simulink model "walkingRobotRL3D"  (R2020b)
settings: Solver=ode23t  StartTime=0.0  StopTime=Tf  RelTol=1e-2  EnableMultiTasking=on
PreLoadFcn:
  | robotParametersRL
undefined symbols (not defined in the file): agent, ankleD_pitch_jointMAX, ankleD_pitch_jointMIN, ankleD_roll_jointMAX, ankleD_roll_jointMIN, ankleI_pitch_jointMAX, ankleI_pitch_jointMIN, ankleI_roll_jointMAX, ankleI_roll_jointMIN, getSampleTime, height_plane, hipD_pitch_jointMAX, hipD_pitch_jointMIN, hipD_roll_jointMAX, hipD_roll_jointMIN, hipI_pitch_jointMAX, hipI_pitch_jointMIN, hipI_roll_jointMAX, hipI_roll_jointMIN, init_angs_L, init_angs_R, init_height, joint_damping, joint_limit_damping, joint_limit_stiffness, joint_stiffness, kneeD_jointMAX, kneeD_jointMIN, kneeI_jointMAX, kneeI_jointMIN, lower_leg_I0, lower_leg_length, lower_leg_mass, lower_leg_x, lower_leg_y, muscle_nominal_length, p10_ankleD_roll, plane_x, plane_y, regulator_type, tau, Tf, torso_height, torso_length, torso_offset_x, torso_offset_z, torso_width, torso_x, torso_y, torso_z, Ts, upper_leg_I0, upper_leg_length, upper_leg_mass, upper_leg_x, upper_leg_y, v10_ankleD_pitch, v10_ankleD_roll, v10_ankleI_pitch, v10_ankleI_roll ... (+41)
libraries: sm_lib x222, simulink x183, nesl_utility x130, walkingRobotUtils x69, rllib x2
(part 15 of 24)

== system walkingRobotRL3D/Walking Robot1/Dynamic model of antagonistic PAM actuators/Spring//Damping (Muscles 2)/Getxmax2 ==
  P2 : Inport
  Bar->kPa : Product
  Constant : Constant  Value=100
  Demux : Demux  Outputs=10
  Mux : Mux  Inputs=10
  getMaxStroke : MATLAB Function  TreatAsAtomicUnit=on
  getMaxStroke1 : MATLAB Function  TreatAsAtomicUnit=on
  getMaxStroke2 : MATLAB Function  TreatAsAtomicUnit=on
  getMaxStroke3 : MATLAB Function  TreatAsAtomicUnit=on
  getMaxStroke4 : MATLAB Function  TreatAsAtomicUnit=on
  getMaxStroke5 : MATLAB Function  TreatAsAtomicUnit=on
  getMaxStroke6 : MATLAB Function  TreatAsAtomicUnit=on
  getMaxStroke7 : MATLAB Function  TreatAsAtomicUnit=on
  getMaxStroke8 : MATLAB Function  TreatAsAtomicUnit=on
  getMaxStroke9 : MATLAB Function  TreatAsAtomicUnit=on
  xmax_muscles2 : Outport
  wires:
  Mux/1 -> xmax_muscles2/1
  P2/1 -> Bar->kPa/2
  Bar->kPa/1 -> Demux/1
  Constant/1 -> Bar->kPa/1
  Demux/1 -> getMaxStroke/1(P2)
  Demux/2 -> getMaxStroke1/1(P2)
  Demux/3 -> getMaxStroke2/1(P2)
  Demux/4 -> getMaxStroke3/1(P2)
  Demux/5 -> getMaxStroke4/1(P2)
  Demux/6 -> getMaxStroke5/1(P2)
  Demux/7 -> getMaxStroke6/1(P2)
  Demux/8 -> getMaxStroke7/1(P2)
  Demux/9 -> getMaxStroke8/1(P2)
  Demux/10 -> getMaxStroke9/1(P2)
  getMaxStroke/1(x_max2) -> Mux/1
  getMaxStroke1/1(x_max2) -> Mux/2
  getMaxStroke2/1(x_max2) -> Mux/3
  getMaxStroke3/1(x_max2) -> Mux/4
  getMaxStroke4/1(x_max2) -> Mux/5
  getMaxStroke5/1(x_max2) -> Mux/6
  getMaxStroke6/1(x_max2) -> Mux/7
  getMaxStroke7/1(x_max2) -> Mux/8
  getMaxStroke8/1(x_max2) -> Mux/9
  getMaxStroke9/1(x_max2) -> Mux/10

== system walkingRobotRL3D/Walking Robot2/Dynamic model of antagonistic PAM actuators/Spring//Damping (Muscles 1)/Get_x1_ankleD_pitch ==
  F1_ankleD_pitchl : Inport
  F2_ankleD_pitch : Inport  Port=2
  S_coef : Inport  Port=3
  Add : Sum  Inputs=+--
  Constant : Constant  Value=tau
  Constant1 : Constant
  Constant2 : Constant  Commented=on  Value=-3.9322
  D_coef : Product
  Divide : Product  Inputs=*/
  IC : InitialCondition  Commented=through  Value=-3.9322
  Integrator : Integrator  InitialCondition=x10_ankleD_pitch
  To Workspace : ToWorkspace  Commented=on  VariableName=S1_ankleD_pitch  SaveFormat=Timeseries  SampleTime=-1
  To Workspace1 : ToWorkspace  Commented=on  VariableName=D1_ankleD_pitch  SaveFormat=Timeseries  SampleTime=-1
  x./D : Product
  xS : Product
  x1_ankleD_pitch : Outport
  wires:
  xS/1 -> Add/3
  x./D/1 -> Integrator/1
  Constant/1 -> D_coef/1
  Divide/1 -> x./D/1
  Constant1/1 -> Divide/1
  D_coef/1 -> To Workspace1/1, Divide/2
  Integrator/1 -> x1_ankleD_pitch/1, xS/1
  IC/1 -> xS/2, To Workspace/1, D_coef/2
  F1_ankleD_pitchl/1 -> Add/1
  F2_ankleD_pitch/1 -> Add/2
  S_coef/1 -> IC/1
  Add/1 -> x./D/2

== system walkingRobotRL3D/Walking Robot2/Dynamic model of antagonistic PAM actuators/Spring//Damping (Muscles 1)/Get_x1_ankleD_roll ==
  F1_ankleD_roll : Inport
  F2_ankleD_roll : Inport  Port=2
  S_coef : Inport  Port=3
  Add : Sum  Inputs=+--
  Constant : Constant  Value=tau
  Constant1 : Constant
  Constant2 : Constant  Commented=on  Value=-3.9322
  D_coef : Product
  Divide : Product  Inputs=*/
  IC : InitialCondition  Commented=through  Value=-3.9322
  Integrator : Integrator  InitialCondition=x10_ankleD_roll
  To Workspace : ToWorkspace  Commented=on  VariableName=S1_ankleD_roll  SaveFormat=Timeseries  SampleTime=-1
  To Workspace1 : ToWorkspace  Commented=on  VariableName=D1_ankleD_roll  SaveFormat=Timeseries  SampleTime=-1
  x./D : Product
  xS : Product
  x1_ankleD_roll : Outport
  wires:
  xS/1 -> Add/3
  x./D/1 -> Integrator/1
  Constant/1 -> D_coef/1
  Divide/1 -> x./D/1
  Constant1/1 -> Divide/1
  D_coef/1 -> To Workspace1/1, Divide/2
  Integrator/1 -> x1_ankleD_roll/1, xS/1
  IC/1 -> xS/2, To Workspace/1, D_coef/2
  F1_ankleD_roll/1 -> Add/1
  F2_ankleD_roll/1 -> Add/2
  S_coef/1 -> IC/1
  Add/1 -> x./D/2

== system walkingRobotRL3D/Walking Robot2/Dynamic model of antagonistic PAM actuators/Spring//Damping (Muscles 1)/Get_x1_ankleI_pitch ==
  F1_ankleI_pitch : Inport
  F2_ankleI_pitch : Inport  Port=2
  S_coef : Inport  Port=3
  Add : Sum  Inputs=+--
  Constant : Constant  Value=tau
  Constant1 : Constant
  D_coef : Product
  Divide : Product  Inputs=*/
  Integrator : Integrator  InitialCondition=x10_ankleI_pitch
  x./D : Product
  xS : Product
  x1_ankleI_pitch : Outport
  wires:
  xS/1 -> Add/3
  Add/1 -> x./D/2
  F1_ankleI_pitch/1 -> Add/1
  F2_ankleI_pitch/1 -> Add/2
  Integrator/1 -> x1_ankleI_pitch/1, xS/1
  S_coef/1 -> D_coef/2, xS/2
  x./D/1 -> Integrator/1
  Constant/1 -> D_coef/1
  Divide/1 -> x./D/1
  Constant1/1 -> Divide/1
  D_coef/1 -> Divide/2

== system walkingRobotRL3D/Walking Robot2/Dynamic model of antagonistic PAM actuators/Spring//Damping (Muscles 1)/Get_x1_ankleI_roll ==
  F1_ankleI_roll : Inport
  F2_ankleI_roll : Inport  Port=2
  S_coef : Inport  Port=3
  Add : Sum  Inputs=+--
  Constant : Constant  Value=tau
  Constant1 : Constant
  D_coef : Product
  Divide : Product  Inputs=*/
  Integrator : Integrator  InitialCondition=x10_ankleI_roll
  x./D : Product
  xS : Product
  x1_ankleI_roll : Outport
  wires:
  xS/1 -> Add/3
  Add/1 -> x./D/2
  F1_ankleI_roll/1 -> Add/1
  F2_ankleI_roll/1 -> Add/2
  Integrator/1 -> x1_ankleI_roll/1, xS/1
  S_coef/1 -> D_coef/2, xS/2
  x./D/1 -> Integrator/1
  Constant/1 -> D_coef/1
  Divide/1 -> x./D/1
  Constant1/1 -> Divide/1
  D_coef/1 -> Divide/2

== system walkingRobotRL3D/Walking Robot2/Dynamic model of antagonistic PAM actuators/Spring//Damping (Muscles 1)/Get_x1_hipD_pitch ==
  F1_hipD_pitch : Inport
  F2_hipD_pitch : Inport  Port=2
  S_coef : Inport  Port=3
  Add : Sum  Inputs=+--
  Constant : Constant  Value=tau
  Constant1 : Constant
  D_coef : Product
  Divide : Product  Inputs=*/
  Integrator : Integrator  InitialCondition=x10_hipD_pitch
  x./D : Product
  xS : Product
  x1_hipD_pitch : Outport
  wires:
  xS/1 -> Add/3
  Add/1 -> x./D/2
  F1_hipD_pitch/1 -> Add/1
  F2_hipD_pitch/1 -> Add/2
  Integrator/1 -> x1_hipD_pitch/1, xS/1
  S_coef/1 -> D_coef/2, xS/2
  x./D/1 -> Integrator/1
  Constant/1 -> D_coef/1
  Divide/1 -> x./D/1
  Constant1/1 -> Divide/1
  D_coef/1 -> Divide/2

== system walkingRobotRL3D/Walking Robot2/Dynamic model of antagonistic PAM actuators/Spring//Damping (Muscles 1)/Get_x1_hipD_roll ==
  F1_hipD_roll : Inport
  F2_hipD_roll : Inport  Port=2
  S_coef : Inport  Port=3
  Add : Sum  Inputs=+--
  Constant : Constant  Value=tau
  Constant1 : Constant
  D_coef : Product
  Divide : Product  Inputs=*/
  Integrator : Integrator  InitialCondition=x10_hipD_roll
  x./D : Product
  xS : Product
  x1_hipD_roll : Outport
  wires:
  xS/1 -> Add/3
  Add/1 -> x./D/2
  F1_hipD_roll/1 -> Add/1
  F2_hipD_roll/1 -> Add/2
  Integrator/1 -> x1_hipD_roll/1, xS/1
  S_coef/1 -> D_coef/2, xS/2
  x./D/1 -> Integrator/1
  Constant/1 -> D_coef/1
  Divide/1 -> x./D/1
  Constant1/1 -> Divide/1
  D_coef/1 -> Divide/2

== system walkingRobotRL3D/Walking Robot2/Dynamic model of antagonistic PAM actuators/Spring//Damping (Muscles 1)/Get_x1_hipI_pitch ==
  F1_hipI_pitch : Inport
  F2_hipI_pitch : Inport  Port=2
  S_coef : Inport  Port=3
  Add : Sum  Inputs=+--
  Constant : Constant  Value=tau
  Constant1 : Constant
  D_coef : Product
  Divide : Product  Inputs=*/
  Integrator : Integrator  InitialCondition=x10_hipI_pitch
  x./D : Product
  xS : Product
  x1_hipI_pitch : Outport
  wires:
  xS/1 -> Add/3
  Add/1 -> x./D/2
  F1_hipI_pitch/1 -> Add/1
  F2_hipI_pitch/1 -> Add/2
  Integrator/1 -> x1_hipI_pitch/1, xS/1
  S_coef/1 -> D_coef/2, xS/2
  x./D/1 -> Integrator/1
  Constant/1 -> D_coef/1
  Divide/1 -> x./D/1
  Constant1/1 -> Divide/1
  D_coef/1 -> Divide/2

== system walkingRobotRL3D/Walking Robot2/Dynamic model of antagonistic PAM actuators/Spring//Damping (Muscles 1)/Get_x1_hipI_roll ==
  F1_hipI_roll : Inport
  F2_hipI_roll : Inport  Port=2
  S_coef : Inport  Port=3
  Add : Sum  Inputs=+--
  Constant : Constant  Value=tau
  Constant1 : Constant
  D_coef : Product
  Divide : Product  Inputs=*/
  Integrator : Integrator  InitialCondition=x10_hipI_roll
  x./D : Product
  xS : Product
  x1_hipI_roll : Outport
  wires:
  xS/1 -> Add/3
  Add/1 -> x./D/2
  F1_hipI_roll/1 -> Add/1
  F2_hipI_roll/1 -> Add/2
  Integrator/1 -> x1_hipI_roll/1, xS/1
  S_coef/1 -> D_coef/2, xS/2
  x./D/1 -> Integrator/1
  Constant/1 -> D_coef/1
  Divide/1 -> x./D/1
  Constant1/1 -> Divide/1
  D_coef/1 -> Divide/2

== system walkingRobotRL3D/Walking Robot2/Dynamic model of antagonistic PAM actuators/Spring//Damping (Muscles 1)/Get_x1_kneeD_1 ==
  F1_kneeD : Inport
  F2_kneeD : Inport  Port=2
  S_coef : Inport  Port=3
  Add : Sum  Inputs=+--
  Constant : Constant  Value=tau
  Constant1 : Constant
  D_coef : Product
  Divide : Product  Inputs=*/
  Integrator : Integrator  InitialCondition=x10_kneeD
  x./D : Product
  xS : Product
  x1_kneeD : Outport
  wires:
  xS/1 -> Add/3
  Add/1 -> x./D/2
  F1_kneeD/1 -> Add/1
  F2_kneeD/1 -> Add/2
  Integrator/1 -> x1_kneeD/1, xS/1
  S_coef/1 -> D_coef/2, xS/2
  x./D/1 -> Integrator/1
  Constant/1 -> D_coef/1
  Divide/1 -> x./D/1
  Constant1/1 -> Divide/1
  D_coef/1 -> Divide/2

== system walkingRobotRL3D/Walking Robot2/Dynamic model of antagonistic PAM actuators/Spring//Damping (Muscles 1)/Get_x1_kneeI ==
  F1_kneeI : Inport
  F2_kneeI : Inport  Port=2
  S_coef : Inport  Port=3
  Add : Sum  Inputs=+--
  Constant : Constant  Value=tau
  Constant1 : Constant
  D_coef : Product
  Divide : Product  Inputs=*/
  Integrator : Integrator  InitialCondition=x10_kneeI
  x./D : Product
  xS : Product
  x1_kneeI : Outport
  wires:
  xS/1 -> Add/3
  Add/1 -> x./D/2
  F1_kneeI/1 -> Add/1
  F2_kneeI/1 -> Add/2
  Integrator/1 -> x1_kneeI/1, xS/1
  S_coef/1 -> D_coef/2, xS/2
  x./D/1 -> Integrator/1
  Constant/1 -> D_coef/1
  Divide/1 -> x./D/1
  Constant1/1 -> Divide/1
  D_coef/1 -> Divide/2

== system walkingRobotRL3D/Walking Robot2/Dynamic model of antagonistic PAM actuators/Spring//Damping (Muscles 1)/Getxmax1 ==
  P1 : Inport
  Bar->kPa : Product
  Constant : Constant  Value=100
  Demux : Demux  Outputs=10
  Mux : Mux  Inputs=10
  To Workspace : ToWorkspace  VariableName=xmax1  SaveFormat=Timeseries  SampleTime=-1
  getMaxStroke : MATLAB Function  TreatAsAtomicUnit=on
  getMaxStroke1 : MATLAB Function  TreatAsAtomicUnit=on
  getMaxStroke2 : MATLAB Function  TreatAsAtomicUnit=on
  getMaxStroke3 : MATLAB Function  TreatAsAtomicUnit=on
  getMaxStroke4 : MATLAB Function  TreatAsAtomicUnit=on
  getMaxStroke5 : MATLAB Function  TreatAsAtomicUnit=on
  getMaxStroke6 : MATLAB Function  TreatAsAtomicUnit=on
  getMaxStroke7 : MATLAB Function  TreatAsAtomicUnit=on
  getMaxStroke8 : MATLAB Function  TreatAsAtomicUnit=on
  getMaxStroke9 : MATLAB Function  TreatAsAtomicUnit=on
  xmax_muscles1 : Outport
  wires:
  Mux/1 -> xmax_muscles1/1
  getMaxStroke/1(x_max1) -> To Workspace/1, Mux/1
  P1/1 -> Bar->kPa/2
  Bar->kPa/1 -> Demux/1
  Constant/1 -> Bar->kPa/1
  Demux/1 -> getMaxStroke/1(P1)
  Demux/2 -> getMaxStroke1/1(P1)
  Demux/3 -> getMaxStroke2/1(P1)
  Demux/4 -> getMaxStroke3/1(P1)
  Demux/5 -> getMaxStroke4/1(P1)
  Demux/6 -> getMaxStroke5/1(P1)
  Demux/7 -> getMaxStroke6/1(P1)
  Demux/8 -> getMaxStroke7/1(P1)
  Demux/9 -> getMaxStroke8/1(P1)
  getMaxStroke1/1(x_max1) -> Mux/2
  getMaxStroke2/1(x_max1) -> Mux/3
  getMaxStroke3/1(x_max1) -> Mux/4
  getMaxStroke4/1(x_max1) -> Mux/5
  getMaxStroke5/1(x_max1) -> Mux/6
  getMaxStroke6/1(x_max1) -> Mux/7
  getMaxStroke7/1(x_max1) -> Mux/8
  getMaxStroke8/1(x_max1) -> Mux/9
  Demux/10 -> getMaxStroke9/1(P1)
  getMaxStroke9/1(x_max1) -> Mux/10

== system walkingRobotRL3D/Walking Robot2/Dynamic model of antagonistic PAM actuators/Spring//Damping (Muscles 2)/Get_x2_ankleD_pitch ==
  F1_ankleD_pitch : Inport
  F2_ankleD_pitch : Inport  Port=2
  S2_coef : Inport  Port=3
  Add : Sum  Inputs=-+-
  Constant : Constant  Value=tau
  Constant1 : Constant
  Constant2 : Constant  Commented=on  Value=3.9338
  D_coef : Product
  Divide : Product  Inputs=*/
  IC : InitialCondition  Commented=through  Value=3.9338
  Integrator : Integrator  InitialCondition=x20_ankleD_pitch
  To Workspace : ToWorkspace  Commented=on  VariableName=S2_ankleD_pitch  SaveFormat=Timeseries  SampleTime=-1
  x./D : Product
  xS : Product
  x2_ankleD_pitch : Outport
  wires:
  xS/1 -> Add/3
  Add/1 -> x./D/2
  F1_ankleD_pitch/1 -> Add/1
  F2_ankleD_pitch/1 -> Add/2
  Integrator/1 -> x2_ankleD_pitch/1, xS/1
  x./D/1 -> Integrator/1
  Constant/1 -> D_coef/1
  Divide/1 -> x./D/1
  Constant1/1 -> Divide/1
  IC/1 -> To Workspace/1, D_coef/2, xS/2
  D_coef/1 -> Divide/2
  S2_coef/1 -> IC/1

== system walkingRobotRL3D/Walking Robot2/Dynamic model of antagonistic PAM actuators/Spring//Damping (Muscles 2)/Get_x2_ankleD_roll ==
  F1_ankleD_roll : Inport
  F2_ankleD_roll : Inport  Port=2
  S2_coef : Inport  Port=3
  Add : Sum  Inputs=-+-
  Constant : Constant  Value=tau
  Constant1 : Constant
  Constant2 : Constant  Commented=on  Value=3.9338
  D_coef : Product
  Divide : Product  Inputs=*/
  IC : InitialCondition  Commented=through  Value=3.9338
  Integrator : Integrator  InitialCondition=x20_ankleD_roll
  To Workspace : ToWorkspace  Commented=on  VariableName=S2_ankleD_roll  SaveFormat=Timeseries  SampleTime=-1
  x./D : Product
  xS : Product
  x2_ankleD_roll : Outport
  wires:
  xS/1 -> Add/3
  Add/1 -> x./D/2
  F1_ankleD_roll/1 -> Add/1
  F2_ankleD_roll/1 -> Add/2
  Integrator/1 -> x2_ankleD_roll/1, xS/1
  x./D/1 -> Integrator/1
  Constant/1 -> D_coef/1
  Divide/1 -> x./D/1
  Constant1/1 -> Divide/1
  IC/1 -> To Workspace/1, D_coef/2, xS/2
  D_coef/1 -> Divide/2
  S2_coef/1 -> IC/1

== system walkingRobotRL3D/Walking Robot2/Dynamic model of antagonistic PAM actuators/Spring//Damping (Muscles 2)/Get_x2_ankleI_pitch ==
  F1_ankleI_pitch : Inport
  F2_ankleI_pitch : Inport  Port=2
  S2_coef : Inport  Port=3
  Add : Sum  Inputs=-+-
  Constant : Constant  Value=tau
  Constant1 : Constant
  D_coef : Product
  Divide : Product  Inputs=*/
  Integrator : Integrator  InitialCondition=x20_ankleI_pitch
  x./D : Product
  xS : Product
  x2_ankleI_pitch : Outport
  wires:
  xS/1 -> Add/3
  Add/1 -> x./D/2
  F1_ankleI_pitch/1 -> Add/1
  F2_ankleI_pitch/1 -> Add/2
  Integrator/1 -> x2_ankleI_pitch/1, xS/1
  S2_coef/1 -> D_coef/2, xS/2
  x./D/1 -> Integrator/1
  Constant/1 -> D_coef/1
  Divide/1 -> x./D/1
  Constant1/1 -> Divide/1
  D_coef/1 -> Divide/2

== system walkingRobotRL3D/Walking Robot2/Dynamic model of antagonistic PAM actuators/Spring//Damping (Muscles 2)/Get_x2_ankleI_roll ==
  F1_ankleI_roll : Inport
  F2_ankleI_roll : Inport  Port=2
  S2_coef : Inport  Port=3
  Add : Sum  Inputs=-+-
  Constant : Constant  Value=tau
  Constant1 : Constant
  D_coef : Product
  Divide : Product  Inputs=*/
  Integrator : Integrator  InitialCondition=x20_ankleI_roll
  x./D : Product
  xS : Product
  x2_ankleI_roll : Outport
  wires:
  xS/1 -> Add/3
  Add/1 -> x./D/2
  F1_ankleI_roll/1 -> Add/1
  F2_ankleI_roll/1 -> Add/2
  Integrator/1 -> x2_ankleI_roll/1, xS/1
  S2_coef/1 -> D_coef/2, xS/2
  x./D/1 -> Integrator/1
  Constant/1 -> D_coef/1
  Divide/1 -> x./D/1
  Constant1/1 -> Divide/1
  D_coef/1 -> Divide/2

== system walkingRobotRL3D/Walking Robot2/Dynamic model of antagonistic PAM actuators/Spring//Damping (Muscles 2)/Get_x2_hipD_pitch ==
  F1_hipD_pitch : Inport
  F2_hipD_pitch : Inport  Port=2
  S2_coef : Inport  Port=3
  Add : Sum  Inputs=-+-
  Constant : Constant  Value=tau
  Constant1 : Constant
  D_coef : Product
  Divide : Product  Inputs=*/
  Integrator : Integrator  InitialCondition=x20_hipD_pitch
  x./D : Product
  xS : Product
  x2_hipD_pitch : Outport
  wires:
  xS/1 -> Add/3
  Add/1 -> x./D/2
  F1_hipD_pitch/1 -> Add/1
  F2_hipD_pitch/1 -> Add/2
  Integrator/1 -> x2_hipD_pitch/1, xS/1
  S2_coef/1 -> D_coef/2, xS/2
  x./D/1 -> Integrator/1
  Constant/1 -> D_coef/1
  Divide/1 -> x./D/1
  Constant1/1 -> Divide/1
  D_coef/1 -> Divide/2

== system walkingRobotRL3D/Walking Robot2/Dynamic model of antagonistic PAM actuators/Spring//Damping (Muscles 2)/Get_x2_hipD_roll ==
  F1_hipD_roll : Inport
  F2_hipD_roll : Inport  Port=2
  S2_coef : Inport  Port=3
  Add : Sum  Inputs=-+-
  Constant : Constant  Value=tau
  Constant1 : Constant
  D_coef : Product
  Divide : Product  Inputs=*/
  Integrator : Integrator  InitialCondition=x20_hipD_roll
  x./D : Product
  xS : Product
  x2_hipD_roll : Outport
  wires:
  xS/1 -> Add/3
  Add/1 -> x./D/2
  F1_hipD_roll/1 -> Add/1
  F2_hipD_roll/1 -> Add/2
  Integrator/1 -> x2_hipD_roll/1, xS/1
  S2_coef/1 -> D_coef/2, xS/2
  x./D/1 -> Integrator/1
  Constant/1 -> D_coef/1
  Divide/1 -> x./D/1
  Constant1/1 -> Divide/1
  D_coef/1 -> Divide/2

== system walkingRobotRL3D/Walking Robot2/Dynamic model of antagonistic PAM actuators/Spring//Damping (Muscles 2)/Get_x2_hipI_pitch ==
  F1_hipI_pitch : Inport
  F2_hipI_pitch : Inport  Port=2
  S2_coef : Inport  Port=3
  Add : Sum  Inputs=-+-
  Constant : Constant  Value=tau
  Constant1 : Constant
  D_coef : Product
  Divide : Product  Inputs=*/
  Integrator : Integrator  InitialCondition=x20_hipI_pitch
  x./D : Product
  xS : Product
  x2_hipI_pitch : Outport
  wires:
  xS/1 -> Add/3
  Add/1 -> x./D/2
  F1_hipI_pitch/1 -> Add/1
  F2_hipI_pitch/1 -> Add/2
  Integrator/1 -> x2_hipI_pitch/1, xS/1
  S2_coef/1 -> D_coef/2, xS/2
  x./D/1 -> Integrator/1
  Constant/1 -> D_coef/1
  Divide/1 -> x./D/1
  Constant1/1 -> Divide/1
  D_coef/1 -> Divide/2

== system walkingRobotRL3D/Walking Robot2/Dynamic model of antagonistic PAM actuators/Spring//Damping (Muscles 2)/Get_x2_hipI_roll ==
  F1_hipI_roll : Inport
  F2_hipI_roll : Inport  Port=2
  S2_coef : Inport  Port=3
  Add : Sum  Inputs=-+-
  Constant : Constant  Value=tau
  Constant1 : Constant
  D_coef : Product
  Divide : Product  Inputs=*/
  Integrator : Integrator  InitialCondition=x20_hipI_roll
  x./D : Product
  xS : Product
  x2_hipI_roll : Outport
  wires:
  xS/1 -> Add/3
  Add/1 -> x./D/2
  F1_hipI_roll/1 -> Add/1
  F2_hipI_roll/1 -> Add/2
  Integrator/1 -> x2_hipI_roll/1, xS/1
  S2_coef/1 -> D_coef/2, xS/2
  x./D/1 -> Integrator/1
  Constant/1 -> D_coef/1
  Divide/1 -> x./D/1
  Constant1/1 -> Divide/1
  D_coef/1 -> Divide/2

== system walkingRobotRL3D/Walking Robot2/Dynamic model of antagonistic PAM actuators/Spring//Damping (Muscles 2)/Get_x2_kneeD ==
  F1_kneeD : Inport
  F2_kneeI : Inport  Port=2
  S2_coef : Inport  Port=3
  Add : Sum  Inputs=-+-
  Constant : Constant  Value=tau
  Constant1 : Constant
  D_coef : Product
  Divide : Product  Inputs=*/
  Integrator : Integrator  InitialCondition=x20_kneeD
  x./D : Product
  xS : Product
  x2_kneeD : Outport
  wires:
  xS/1 -> Add/3
  Add/1 -> x./D/2
  F1_kneeD/1 -> Add/1
  F2_kneeI/1 -> Add/2
  Integrator/1 -> x2_kneeD/1, xS/1
  S2_coef/1 -> D_coef/2, xS/2
  x./D/1 -> Integrator/1
  Constant/1 -> D_coef/1
  Divide/1 -> x./D/1
  Constant1/1 -> Divide/1
  D_coef/1 -> Divide/2

== system walkingRobotRL3D/Walking Robot2/Dynamic model of antagonistic PAM actuators/Spring//Damping (Muscles 2)/Get_x2_kneeI ==
  F1_kneeI : Inport
  F2_kneeI : Inport  Port=2
  S2_coef : Inport  Port=3
  Add : Sum  Inputs=-+-
  Constant : Constant  Value=tau
  Constant1 : Constant
  D_coef : Product
  Divide : Product  Inputs=*/
  Integrator : Integrator  InitialCondition=x20_kneeI
  x./D : Product
  xS : Product
  x2_kneeI : Outport
  wires:
  xS/1 -> Add/3
  Add/1 -> x./D/2
  F1_kneeI/1 -> Add/1
  F2_kneeI/1 -> Add/2
  Integrator/1 -> x2_kneeI/1, xS/1
  S2_coef/1 -> D_coef/2, xS/2
  x./D/1 -> Integrator/1
  Constant/1 -> D_coef/1
  Divide/1 -> x./D/1
  Constant1/1 -> Divide/1
  D_coef/1 -> Divide/2

== system walkingRobotRL3D/Walking Robot2/Dynamic model of antagonistic PAM actuators/Spring//Damping (Muscles 2)/Getxmax2 ==
  P2 : Inport
  Bar->kPa : Product
  Constant : Constant  Value=100
  Demux : Demux  Outputs=10
  Mux : Mux  Inputs=10
  getMaxStroke : MATLAB Function  TreatAsAtomicUnit=on
  getMaxStroke1 : MATLAB Function  TreatAsAtomicUnit=on
  getMaxStroke2 : MATLAB Function  TreatAsAtomicUnit=on
  getMaxStroke3 : MATLAB Function  TreatAsAtomicUnit=on
  getMaxStroke4 : MATLAB Function  TreatAsAtomicUnit=on
  getMaxStroke5 : MATLAB Function  TreatAsAtomicUnit=on
  getMaxStroke6 : MATLAB Function  TreatAsAtomicUnit=on
  getMaxStroke7 : MATLAB Function  TreatAsAtomicUnit=on
  getMaxStroke8 : MATLAB Function  TreatAsAtomicUnit=on
  getMaxStroke9 : MATLAB Function  TreatAsAtomicUnit=on
  xmax_muscles2 : Outport
  wires:
  Mux/1 -> xmax_muscles2/1
  P2/1 -> Bar->kPa/2
  Bar->kPa/1 -> Demux/1
  Constant/1 -> Bar->kPa/1
  Demux/1 -> getMaxStroke/1(P2)
  Demux/2 -> getMaxStroke1/1(P2)
  Demux/3 -> getMaxStroke2/1(P2)
  Demux/4 -> getMaxStroke3/1(P2)
  Demux/5 -> getMaxStroke4/1(P2)
  Demux/6 -> getMaxStroke5/1(P2)
  Demux/7 -> getMaxStroke6/1(P2)
  Demux/8 -> getMaxStroke7/1(P2)
  Demux/9 -> getMaxStroke8/1(P2)
  Demux/10 -> getMaxStroke9/1(P2)
  getMaxStroke/1(x_max2) -> Mux/1
  getMaxStroke1/1(x_max2) -> Mux/2
  getMaxStroke2/1(x_max2) -> Mux/3
  getMaxStroke3/1(x_max2) -> Mux/4
  getMaxStroke4/1(x_max2) -> Mux/5
  getMaxStroke5/1(x_max2) -> Mux/6
  getMaxStroke6/1(x_max2) -> Mux/7
  getMaxStroke7/1(x_max2) -> Mux/8
  getMaxStroke8/1(x_max2) -> Mux/9
  getMaxStroke9/1(x_max2) -> Mux/10

== system walkingRobotRL3D/Walking Robot33/DYNAMIC MODEL OF PAM FOR LEFT LEG/Dynamic Model Antagonisitic PAM1/Spring and damping model ==
  F1 : Inport
  F2 : Inport  Port=2
  P1 : Inport  Port=3
  P2 : Inport  Port=4
  Dynamic muscle 2 : Subsystem
  Dynamics muscle 1 : Subsystem
  S(P),D(P) : MATLAB Function  TreatAsAtomicUnit=on
  Unit Delay : UnitDelay  SampleTime=-1  HasFrameUpgradeWarning=on
  Unit Delay1 : UnitDelay  SampleTime=-1  HasFrameUpgradeWarning=on
  Unit Delay2 : UnitDelay  Commented=through  SampleTime=-1  HasFrameUpgradeWarning=on
  Unit Delay3 : UnitDelay  Commented=through  SampleTime=-1  HasFrameUpgradeWarning=on
  x1(m)->x1(%) : Gain  Gain=100/muscle_nominal_length
  x2(m)->x2(%) : Gain  Gain=100/muscle_nominal_length
  x2 : Outport
  x1 : Outport  Port=2
  wires:
  Dynamics muscle 1/1(R1) -> Unit Delay/1
  F1/1 -> Unit Delay2/1
  Dynamic muscle 2/2(x2) -> x2(m)->x2(%)/1
  Dynamics muscle 1/2(x1) -> x1(m)->x1(%)/1
  P1/1 -> S(P),D(P)/1(P1)
  x2(m)->x2(%)/1 -> x2/1
  x1(m)->x1(%)/1 -> x1/1
  F2/1 -> Unit Delay3/1
  P2/1 -> S(P),D(P)/2(P2)
  Unit Delay/1 -> Dynamic muscle 2/2(R1)
  Dynamic muscle 2/1(R2) -> Unit Delay1/1
  Unit Delay1/1 -> Dynamics muscle 1/3(R2)
  Unit Delay2/1 -> Dynamics muscle 1/1(F1)
  Unit Delay3/1 -> Dynamic muscle 2/3(F2)
  S(P),D(P)/2(D1) -> Dynamics muscle 1/4(D1)
  S(P),D(P)/3(S2) -> Dynamic muscle 2/1(S2)
  S(P),D(P)/4(D2) -> Dynamic muscle 2/4(D2)
  S(P),D(P)/1(S1) -> Dynamics muscle 1/2(S1)

== system walkingRobotRL3D/Walking Robot33/DYNAMIC MODEL OF PAM FOR LEFT LEG/Dynamic Model Antagonisitic PAM2/Spring and damping model ==
  F1 : Inport
  F2 : Inport  Port=2
  P1 : Inport  Port=3
  P2 : Inport  Port=4
  Dynamic muscle 2 : Subsystem
  Dynamics muscle 1 : Subsystem
  S(P),D(P) : MATLAB Function  TreatAsAtomicUnit=on
  Unit Delay : UnitDelay  SampleTime=-1  HasFrameUpgradeWarning=on
  Unit Delay1 : UnitDelay  SampleTime=-1  HasFrameUpgradeWarning=on
  Unit Delay2 : UnitDelay  Commented=through  SampleTime=-1  HasFrameUpgradeWarning=on
  Unit Delay3 : UnitDelay  Commented=through  SampleTime=-1  HasFrameUpgradeWarning=on
  x1(m)->x1(%) : Gain  Gain=100/muscle_nominal_length
  x2(m)->x2(%) : Gain  Gain=100/muscle_nominal_length
  x2 : Outport
  x1 : Outport  Port=2
  wires:
  Dynamics muscle 1/1(R1) -> Unit Delay/1
  F1/1 -> Unit Delay2/1
  Dynamic muscle 2/2(x2) -> x2(m)->x2(%)/1
  Dynamics muscle 1/2(x1) -> x1(m)->x1(%)/1
  P1/1 -> S(P),D(P)/1(P1)
  x2(m)->x2(%)/1 -> x2/1
  x1(m)->x1(%)/1 -> x1/1
  F2/1 -> Unit Delay3/1
  P2/1 -> S(P),D(P)/2(P2)
  Unit Delay/1 -> Dynamic muscle 2/2(R1)
  Dynamic muscle 2/1(R2) -> Unit Delay1/1
  Unit Delay1/1 -> Dynamics muscle 1/3(R2)
  Unit Delay2/1 -> Dynamics muscle 1/1(F1)
  Unit Delay3/1 -> Dynamic muscle 2/3(F2)
  S(P),D(P)/2(D1) -> Dynamics muscle 1/4(D1)
  S(P),D(P)/3(S2) -> Dynamic muscle 2/1(S2)
  S(P),D(P)/4(D2) -> Dynamic muscle 2/4(D2)
  S(P),D(P)/1(S1) -> Dynamics muscle 1/2(S1)

== system walkingRobotRL3D/Walking Robot33/DYNAMIC MODEL OF PAM FOR LEFT LEG/Dynamic Model Antagonisitic PAM3/Spring and damping model ==
  F1 : Inport
  F2 : Inport  Port=2
  P1 : Inport  Port=3
  P2 : Inport  Port=4
  Dynamic muscle 2 : Subsystem
  Dynamics muscle 1 : Subsystem
  S(P),D(P) : MATLAB Function  TreatAsAtomicUnit=on
  Unit Delay : UnitDelay  SampleTime=-1  HasFrameUpgradeWarning=on
  Unit Delay1 : UnitDelay  SampleTime=-1  HasFrameUpgradeWarning=on
  Unit Delay2 : UnitDelay  Commented=through  SampleTime=-1  HasFrameUpgradeWarning=on
  Unit Delay3 : UnitDelay  Commented=through  SampleTime=-1  HasFrameUpgradeWarning=on
  x1(m)->x1(%) : Gain  Gain=100/muscle_nominal_length
  x2(m)->x2(%) : Gain  Gain=100/muscle_nominal_length
  x2 : Outport
  x1 : Outport  Port=2
  wires:
  Dynamics muscle 1/1(R1) -> Unit Delay/1
  F1/1 -> Unit Delay2/1
  Dynamic muscle 2/2(x2) -> x2(m)->x2(%)/1
  Dynamics muscle 1/2(x1) -> x1(m)->x1(%)/1
  P1/1 -> S(P),D(P)/1(P1)
  x2(m)->x2(%)/1 -> x2/1
  x1(m)->x1(%)/1 -> x1/1
  F2/1 -> Unit Delay3/1
  P2/1 -> S(P),D(P)/2(P2)
  Unit Delay/1 -> Dynamic muscle 2/2(R1)
  Dynamic muscle 2/1(R2) -> Unit Delay1/1
  Unit Delay1/1 -> Dynamics muscle 1/3(R2)
  Unit Delay2/1 -> Dynamics muscle 1/1(F1)
  Unit Delay3/1 -> Dynamic muscle 2/3(F2)
  S(P),D(P)/2(D1) -> Dynamics muscle 1/4(D1)
  S(P),D(P)/3(S2) -> Dynamic muscle 2/1(S2)
  S(P),D(P)/4(D2) -> Dynamic muscle 2/4(D2)
  S(P),D(P)/1(S1) -> Dynamics muscle 1/2(S1)

== system walkingRobotRL3D/Walking Robot33/DYNAMIC MODEL OF PAM FOR LEFT LEG/Dynamic Model Antagonisitic PAM4/Spring and damping model ==
  F1 : Inport
  F2 : Inport  Port=2
  P1 : Inport  Port=3
  P2 : Inport  Port=4
  Dynamic muscle 2 : Subsystem
  Dynamics muscle 1 : Subsystem
  S(P),D(P) : MATLAB Function  TreatAsAtomicUnit=on
  Unit Delay : UnitDelay  SampleTime=-1  HasFrameUpgradeWarning=on
  Unit Delay1 : UnitDelay  SampleTime=-1  HasFrameUpgradeWarning=on
  Unit Delay2 : UnitDelay  Commented=through  SampleTime=-1  HasFrameUpgradeWarning=on
  Unit Delay3 : UnitDelay  Commented=through  SampleTime=-1  HasFrameUpgradeWarning=on
  x1(m)->x1(%) : Gain  Gain=100/muscle_nominal_length
  x2(m)->x2(%) : Gain  Gain=100/muscle_nominal_length
  x2 : Outport
  x1 : Outport  Port=2
  wires:
  Dynamics muscle 1/1(R1) -> Unit Delay/1
  F1/1 -> Unit Delay2/1
  Dynamic muscle 2/2(x2) -> x2(m)->x2(%)/1
  Dynamics muscle 1/2(x1) -> x1(m)->x1(%)/1
  P1/1 -> S(P),D(P)/1(P1)
  x2(m)->x2(%)/1 -> x2/1
  x1(m)->x1(%)/1 -> x1/1
  F2/1 -> Unit Delay3/1
  P2/1 -> S(P),D(P)/2(P2)
  Unit Delay/1 -> Dynamic muscle 2/2(R1)
  Dynamic muscle 2/1(R2) -> Unit Delay1/1
  Unit Delay1/1 -> Dynamics muscle 1/3(R2)
  Unit Delay2/1 -> Dynamics muscle 1/1(F1)
  Unit Delay3/1 -> Dynamic muscle 2/3(F2)
  S(P),D(P)/2(D1) -> Dynamics muscle 1/4(D1)
  S(P),D(P)/3(S2) -> Dynamic muscle 2/1(S2)
  S(P),D(P)/4(D2) -> Dynamic muscle 2/4(D2)
  S(P),D(P)/1(S1) -> Dynamics muscle 1/2(S1)

== system walkingRobotRL3D/Walking Robot33/DYNAMIC MODEL OF PAM FOR LEFT LEG/Dynamic Model Antagonisitic PAM5/Spring and damping model ==
  F1 : Inport
  F2 : Inport  Port=2
  P1 : Inport  Port=3
  P2 : Inport  Port=4
  Dynamic muscle 2 : Subsystem
  Dynamics muscle 1 : Subsystem
  S(P),D(P) : MATLAB Function  TreatAsAtomicUnit=on
  Unit Delay : UnitDelay  SampleTime=-1  HasFrameUpgradeWarning=on
  Unit Delay1 : UnitDelay  SampleTime=-1  HasFrameUpgradeWarning=on
  Unit Delay2 : UnitDelay  Commented=through  SampleTime=-1  HasFrameUpgradeWarning=on
  Unit Delay3 : UnitDelay  Commented=through  SampleTime=-1  HasFrameUpgradeWarning=on
  x1(m)->x1(%) : Gain  Gain=100/muscle_nominal_length
  x2(m)->x2(%) : Gain  Gain=100/muscle_nominal_length
  x2 : Outport
  x1 : Outport  Port=2
  wires:
  Dynamics muscle 1/1(R1) -> Unit Delay/1
  F1/1 -> Unit Delay2/1
  Dynamic muscle 2/2(x2) -> x2(m)->x2(%)/1
  Dynamics muscle 1/2(x1) -> x1(m)->x1(%)/1
  P1/1 -> S(P),D(P)/1(P1)
  x2(m)->x2(%)/1 -> x2/1
  x1(m)->x1(%)/1 -> x1/1
  F2/1 -> Unit Delay3/1
  P2/1 -> S(P),D(P)/2(P2)
  Unit Delay/1 -> Dynamic muscle 2/2(R1)
  Dynamic muscle 2/1(R2) -> Unit Delay1/1
  Unit Delay1/1 -> Dynamics muscle 1/3(R2)
  Unit Delay2/1 -> Dynamics muscle 1/1(F1)
  Unit Delay3/1 -> Dynamic muscle 2/3(F2)
  S(P),D(P)/2(D1) -> Dynamics muscle 1/4(D1)
  S(P),D(P)/3(S2) -> Dynamic muscle 2/1(S2)
  S(P),D(P)/4(D2) -> Dynamic muscle 2/4(D2)
  S(P),D(P)/1(S1) -> Dynamics muscle 1/2(S1)

== system walkingRobotRL3D/Walking Robot33/DYNAMIC MODEL OF PAM FOR RIGHT LEG/Dynamic Model Antagonisitic PAM1/Spring and damping model ==
  F1 : Inport
  F2 : Inport  Port=2
  P1 : Inport  Port=3
  P2 : Inport  Port=4
  Dynamic muscle 2 : Subsystem
  Dynamics muscle 1 : Subsystem
  S(P),D(P) : MATLAB Function  TreatAsAtomicUnit=on
  Unit Delay : UnitDelay  SampleTime=-1  HasFrameUpgradeWarning=on
  Unit Delay1 : UnitDelay  SampleTime=-1  HasFrameUpgradeWarning=on
  Unit Delay2 : UnitDelay  Commented=through  SampleTime=-1  HasFrameUpgradeWarning=on
  Unit Delay3 : UnitDelay  Commented=through  SampleTime=-1  HasFrameUpgradeWarning=on
  x1(m)->x1(%) : Gain  Gain=100/muscle_nominal_length
  x2(m)->x2(%) : Gain  Gain=100/muscle_nominal_length
  x2 : Outport
  x1 : Outport  Port=2
  wires:
  Dynamics muscle 1/1(R1) -> Unit Delay/1
  F1/1 -> Unit Delay2/1
  Dynamic muscle 2/2(x2) -> x2(m)->x2(%)/1
  Dynamics muscle 1/2(x1) -> x1(m)->x1(%)/1
  P1/1 -> S(P),D(P)/1(P1)
  x2(m)->x2(%)/1 -> x2/1
  x1(m)->x1(%)/1 -> x1/1
  F2/1 -> Unit Delay3/1
  P2/1 -> S(P),D(P)/2(P2)
  Unit Delay/1 -> Dynamic muscle 2/2(R1)
  Dynamic muscle 2/1(R2) -> Unit Delay1/1
  Unit Delay1/1 -> Dynamics muscle 1/3(R2)
  Unit Delay2/1 -> Dynamics muscle 1/1(F1)
  Unit Delay3/1 -> Dynamic muscle 2/3(F2)
  S(P),D(P)/2(D1) -> Dynamics muscle 1/4(D1)
  S(P),D(P)/3(S2) -> Dynamic muscle 2/1(S2)
  S(P),D(P)/4(D2) -> Dynamic muscle 2/4(D2)
  S(P),D(P)/1(S1) -> Dynamics muscle 1/2(S1)

== system walkingRobotRL3D/Walking Robot33/DYNAMIC MODEL OF PAM FOR RIGHT LEG/Dynamic Model Antagonisitic PAM2/Spring and damping model ==
  F1 : Inport
  F2 : Inport  Port=2
  P1 : Inport  Port=3
  P2 : Inport  Port=4
  Dynamic muscle 2 : Subsystem
  Dynamics muscle 1 : Subsystem
  S(P),D(P) : MATLAB Function  TreatAsAtomicUnit=on
  Unit Delay : UnitDelay  SampleTime=-1  HasFrameUpgradeWarning=on
  Unit Delay1 : UnitDelay  SampleTime=-1  HasFrameUpgradeWarning=on
  Unit Delay2 : UnitDelay  Commented=through  SampleTime=-1  HasFrameUpgradeWarning=on
  Unit Delay3 : UnitDelay  Commented=through  SampleTime=-1  HasFrameUpgradeWarning=on
  x1(m)->x1(%) : Gain  Gain=100/muscle_nominal_length
  x2(m)->x2(%) : Gain  Gain=100/muscle_nominal_length
  x2 : Outport
  x1 : Outport  Port=2
  wires:
  Dynamics muscle 1/1(R1) -> Unit Delay/1
  F1/1 -> Unit Delay2/1
  Dynamic muscle 2/2(x2) -> x2(m)->x2(%)/1
  Dynamics muscle 1/2(x1) -> x1(m)->x1(%)/1
  P1/1 -> S(P),D(P)/1(P1)
  x2(m)->x2(%)/1 -> x2/1
  x1(m)->x1(%)/1 -> x1/1
  F2/1 -> Unit Delay3/1
  P2/1 -> S(P),D(P)/2(P2)
  Unit Delay/1 -> Dynamic muscle 2/2(R1)
  Dynamic muscle 2/1(R2) -> Unit Delay1/1
  Unit Delay1/1 -> Dynamics muscle 1/3(R2)
  Unit Delay2/1 -> Dynamics muscle 1/1(F1)
  Unit Delay3/1 -> Dynamic muscle 2/3(F2)
  S(P),D(P)/2(D1) -> Dynamics muscle 1/4(D1)
  S(P),D(P)/3(S2) -> Dynamic muscle 2/1(S2)
  S(P),D(P)/4(D2) -> Dynamic muscle 2/4(D2)
  S(P),D(P)/1(S1) -> Dynamics muscle 1/2(S1)

== system walkingRobotRL3D/Walking Robot33/DYNAMIC MODEL OF PAM FOR RIGHT LEG/Dynamic Model Antagonisitic PAM3/Spring and damping model ==
  F1 : Inport
  F2 : Inport  Port=2
  P1 : Inport  Port=3
  P2 : Inport  Port=4
  Dynamic muscle 2 : Subsystem
  Dynamics muscle 1 : Subsystem
  S(P),D(P) : MATLAB Function  TreatAsAtomicUnit=on
  Unit Delay : UnitDelay  SampleTime=-1  HasFrameUpgradeWarning=on
  Unit Delay1 : UnitDelay  SampleTime=-1  HasFrameUpgradeWarning=on
  Unit Delay2 : UnitDelay  Commented=through  SampleTime=-1  HasFrameUpgradeWarning=on
  Unit Delay3 : UnitDelay  Commented=through  SampleTime=-1  HasFrameUpgradeWarning=on
  x1(m)->x1(%) : Gain  Gain=100/muscle_nominal_length
  x2(m)->x2(%) : Gain  Gain=100/muscle_nominal_length
  x2 : Outport
  x1 : Outport  Port=2
  wires:
  Dynamics muscle 1/1(R1) -> Unit Delay/1
  F1/1 -> Unit Delay2/1
  Dynamic muscle 2/2(x2) -> x2(m)->x2(%)/1
  Dynamics muscle 1/2(x1) -> x1(m)->x1(%)/1
  P1/1 -> S(P),D(P)/1(P1)
  x2(m)->x2(%)/1 -> x2/1
  x1(m)->x1(%)/1 -> x1/1
  F2/1 -> Unit Delay3/1
  P2/1 -> S(P),D(P)/2(P2)
  Unit Delay/1 -> Dynamic muscle 2/2(R1)
  Dynamic muscle 2/1(R2) -> Unit Delay1/1
  Unit Delay1/1 -> Dynamics muscle 1/3(R2)
  Unit Delay2/1 -> Dynamics muscle 1/1(F1)
  Unit Delay3/1 -> Dynamic muscle 2/3(F2)
  S(P),D(P)/2(D1) -> Dynamics muscle 1/4(D1)
  S(P),D(P)/3(S2) -> Dynamic muscle 2/1(S2)
  S(P),D(P)/4(D2) -> Dynamic muscle 2/4(D2)
  S(P),D(P)/1(S1) -> Dynamics muscle 1/2(S1)

== system walkingRobotRL3D/Walking Robot33/DYNAMIC MODEL OF PAM FOR RIGHT LEG/Dynamic Model Antagonisitic PAM4/Spring and damping model ==
  F1 : Inport
  F2 : Inport  Port=2
  P1 : Inport  Port=3
  P2 : Inport  Port=4
  Dynamic muscle 2 : Subsystem
  Dynamics muscle 1 : Subsystem
  S(P),D(P) : MATLAB Function  TreatAsAtomicUnit=on
  Unit Delay : UnitDelay  SampleTime=-1  HasFrameUpgradeWarning=on
  Unit Delay1 : UnitDelay  SampleTime=-1  HasFrameUpgradeWarning=on
  Unit Delay2 : UnitDelay  Commented=through  SampleTime=-1  HasFrameUpgradeWarning=on
  Unit Delay3 : UnitDelay  Commented=through  SampleTime=-1  HasFrameUpgradeWarning=on
  x1(m)->x1(%) : Gain  Gain=100/muscle_nominal_length
  x2(m)->x2(%) : Gain  Gain=100/muscle_nominal_length
  x2 : Outport
  x1 : Outport  Port=2
  wires:
  Dynamics muscle 1/1(R1) -> Unit Delay/1
  F1/1 -> Unit Delay2/1
  Dynamic muscle 2/2(x2) -> x2(m)->x2(%)/1
  Dynamics muscle 1/2(x1) -> x1(m)->x1(%)/1
  P1/1 -> S(P),D(P)/1(P1)
  x2(m)->x2(%)/1 -> x2/1
  x1(m)->x1(%)/1 -> x1/1
  F2/1 -> Unit Delay3/1
  P2/1 -> S(P),D(P)/2(P2)
  Unit Delay/1 -> Dynamic muscle 2/2(R1)
  Dynamic muscle 2/1(R2) -> Unit Delay1/1
  Unit Delay1/1 -> Dynamics muscle 1/3(R2)
  Unit Delay2/1 -> Dynamics muscle 1/1(F1)
  Unit Delay3/1 -> Dynamic muscle 2/3(F2)
  S(P),D(P)/2(D1) -> Dynamics muscle 1/4(D1)
  S(P),D(P)/3(S2) -> Dynamic muscle 2/1(S2)
  S(P),D(P)/4(D2) -> Dynamic muscle 2/4(D2)
  S(P),D(P)/1(S1) -> Dynamics muscle 1/2(S1)

== system walkingRobotRL3D/Walking Robot33/DYNAMIC MODEL OF PAM FOR RIGHT LEG/Dynamic Model Antagonisitic PAM5/Spring and damping model ==
  F1 : Inport
  F2 : Inport  Port=2
  P1 : Inport  Port=3
  P2 : Inport  Port=4
  Dynamic muscle 2 : Subsystem
  Dynamics muscle 1 : Subsystem
  S(P),D(P) : MATLAB Function  TreatAsAtomicUnit=on
  Unit Delay : UnitDelay  SampleTime=-1  HasFrameUpgradeWarning=on
  Unit Delay1 : UnitDelay  SampleTime=-1  HasFrameUpgradeWarning=on
  Unit Delay2 : UnitDelay  Commented=through  SampleTime=-1  HasFrameUpgradeWarning=on
  Unit Delay3 : UnitDelay  Commented=through  SampleTime=-1  HasFrameUpgradeWarning=on
  x1(m)->x1(%) : Gain  Gain=100/muscle_nominal_length
  x2(m)->x2(%) : Gain  Gain=100/muscle_nominal_length
  x2 : Outport
  x1 : Outport  Port=2
  wires:
  Dynamics muscle 1/1(R1) -> Unit Delay/1
  F1/1 -> Unit Delay2/1
  Dynamic muscle 2/2(x2) -> x2(m)->x2(%)/1
  Dynamics muscle 1/2(x1) -> x1(m)->x1(%)/1
  P1/1 -> S(P),D(P)/1(P1)
  x2(m)->x2(%)/1 -> x2/1
  x1(m)->x1(%)/1 -> x1/1
  F2/1 -> Unit Delay3/1
  P2/1 -> S(P),D(P)/2(P2)
  Unit Delay/1 -> Dynamic muscle 2/2(R1)
  Dynamic muscle 2/1(R2) -> Unit Delay1/1
  Unit Delay1/1 -> Dynamics muscle 1/3(R2)
  Unit Delay2/1 -> Dynamics muscle 1/1(F1)
  Unit Delay3/1 -> Dynamic muscle 2/3(F2)
  S(P),D(P)/2(D1) -> Dynamics muscle 1/4(D1)
  S(P),D(P)/3(S2) -> Dynamic muscle 2/1(S2)
  S(P),D(P)/4(D2) -> Dynamic muscle 2/4(D2)
  S(P),D(P)/1(S1) -> Dynamics muscle 1/2(S1)

== system walkingRobotRL3D/Walking Robot/DYNAMIC MODEL OF PAM FOR LEFT LEG/Dynamic Model Antagonisitic PAM1/Spring and damping model/Dynamic muscle 2 ==
  S2 : Inport
  R1 : Inport  Port=2
  F2 : Inport  Port=3
  D2 : Inport  Port=4
  Add : Sum  Inputs=+--
  Add1 : Sum  Inputs=+--
  Constant3 : Constant
  Divide1 : Product  Inputs=*/
  Integrator1 : Integrator  InitialCondition=x20_ankleI_pitch
  Unit Delay : UnitDelay  Commented=through  SampleTime=-1  HasFrameUpgradeWarning=on
  Unit Delay1 : UnitDelay  Commented=through  SampleTime=-1  HasFrameUpgradeWarning=on
  Unit Delay2 : UnitDelay  Commented=through  SampleTime=-1  HasFrameUpgradeWarning=on
  x./D2 : Product
  xS2 : Product
  R2 : Outport
  x2 : Outport  Port=2
  wires:
  F2/1 -> Unit Delay1/1, Add1/1
  Divide1/1 -> x./D2/1
  Integrator1/1 -> x2/1, xS2/1
  x./D2/1 -> Integrator1/1
  Add1/1 -> Unit Delay/1, x./D2/2
  Constant3/1 -> Divide1/1
  R1/1 -> Add1/2
  S2/1 -> xS2/2
  Add/1 -> R2/1
  Unit Delay/1 -> Add/3
  xS2/1 -> Unit Delay2/1, Add1/3
  Unit Delay1/1 -> Add/1
  Unit Delay2/1 -> Add/2
  D2/1 -> Divide1/2

== system walkingRobotRL3D/Walking Robot/DYNAMIC MODEL OF PAM FOR LEFT LEG/Dynamic Model Antagonisitic PAM1/Spring and damping model/Dynamics muscle 1 ==
  F1 : Inport
  S1 : Inport  Port=2
  R2 : Inport  Port=3
  D1 : Inport  Port=4
  Add : Sum  Inputs=+--
  Add1 : Sum  Inputs=+--
  Constant1 : Constant
  Divide : Product  Inputs=*/
  Integrator : Integrator  InitialCondition=x10_ankleI_pitch
  Unit Delay : UnitDelay  Commented=through  SampleTime=-1  HasFrameUpgradeWarning=on
  Unit Delay1 : UnitDelay  Commented=through  SampleTime=-1  HasFrameUpgradeWarning=on
  Unit Delay2 : UnitDelay  Commented=through  SampleTime=-1  HasFrameUpgradeWarning=on
  x./D1 : Product
  xS1 : Product
  R1 : Outport
  x1 : Outport  Port=2
  wires:
  Integrator/1 -> xS1/1, x1/1
  Divide/1 -> x./D1/1
  F1/1 -> Unit Delay1/1, Add/1
  x./D1/1 -> Integrator/1
  Add/1 -> Unit Delay/1, x./D1/2
  S1/1 -> xS1/2
  Constant1/1 -> Divide/1
  R2/1 -> Add/2
  Unit Delay/1 -> Add1/3
  Add1/1 -> R1/1
  xS1/1 -> Unit Delay2/1, Add/3
  D1/1 -> Divide/2
  Unit Delay1/1 -> Add1/1
  Unit Delay2/1 -> Add1/2

== system walkingRobotRL3D/Walking Robot/DYNAMIC MODEL OF PAM FOR LEFT LEG/Dynamic Model Antagonisitic PAM2/Spring and damping model/Dynamic muscle 2 ==
  S2 : Inport
  R1 : Inport  Port=2
  F2 : Inport  Port=3
  D2 : Inport  Port=4
  Add : Sum  Inputs=+--
  Add1 : Sum  Inputs=+--
  Constant3 : Constant
  Divide1 : Product  Inputs=*/
  Integrator1 : Integrator  InitialCondition=x20_kneeI
  Unit Delay : UnitDelay  Commented=through  SampleTime=-1  HasFrameUpgradeWarning=on
  Unit Delay1 : UnitDelay  Commented=through  SampleTime=-1  HasFrameUpgradeWarning=on
  Unit Delay2 : UnitDelay  Commented=through  SampleTime=-1  HasFrameUpgradeWarning=on
  x./D2 : Product
  xS2 : Product
  R2 : Outport
  x2 : Outport  Port=2
  wires:
  F2/1 -> Unit Delay1/1, Add1/1
  Divide1/1 -> x./D2/1
  Integrator1/1 -> x2/1, xS2/1
  x./D2/1 -> Integrator1/1
  Add1/1 -> Unit Delay/1, x./D2/2
  Constant3/1 -> Divide1/1
  R1/1 -> Add1/2
  S2/1 -> xS2/2
  Add/1 -> R2/1
  Unit Delay/1 -> Add/3
  xS2/1 -> Unit Delay2/1, Add1/3
  Unit Delay1/1 -> Add/1
  Unit Delay2/1 -> Add/2
  D2/1 -> Divide1/2

== system walkingRobotRL3D/Walking Robot/DYNAMIC MODEL OF PAM FOR LEFT LEG/Dynamic Model Antagonisitic PAM2/Spring and damping model/Dynamics muscle 1 ==
  F1 : Inport
  S1 : Inport  Port=2
  R2 : Inport  Port=3
  D1 : Inport  Port=4
  Add : Sum  Inputs=+--
  Add1 : Sum  Inputs=+--
  Constant1 : Constant
  Divide : Product  Inputs=*/
  Integrator : Integrator  InitialCondition=x10_kneeI
  Unit Delay : UnitDelay  Commented=through  SampleTime=-1  HasFrameUpgradeWarning=on
  Unit Delay1 : UnitDelay  Commented=through  SampleTime=-1  HasFrameUpgradeWarning=on
  Unit Delay2 : UnitDelay  Commented=through  SampleTime=-1  HasFrameUpgradeWarning=on
  x./D1 : Product
  xS1 : Product
  R1 : Outport
  x1 : Outport  Port=2
  wires:
  Integrator/1 -> xS1/1, x1/1
  Divide/1 -> x./D1/1
  F1/1 -> Unit Delay1/1, Add/1
  x./D1/1 -> Integrator/1
  Add/1 -> Unit Delay/1, x./D1/2
  S1/1 -> xS1/2
  Constant1/1 -> Divide/1
  R2/1 -> Add/2
  Unit Delay/1 -> Add1/3
  Add1/1 -> R1/1
  xS1/1 -> Unit Delay2/1, Add/3
  D1/1 -> Divide/2
  Unit Delay1/1 -> Add1/1
  Unit Delay2/1 -> Add1/2

== system walkingRobotRL3D/Walking Robot/DYNAMIC MODEL OF PAM FOR LEFT LEG/Dynamic Model Antagonisitic PAM3/Spring and damping model/Dynamic muscle 2 ==
  S2 : Inport
  R1 : Inport  Port=2
  F2 : Inport  Port=3
  D2 : Inport  Port=4
  Add : Sum  Inputs=+--
  Add1 : Sum  Inputs=+--
  Constant3 : Constant
  Divide1 : Product  Inputs=*/
  Integrator1 : Integrator  InitialCondition=x20_ankleI_roll
  Unit Delay : UnitDelay  Commented=through  SampleTime=-1  HasFrameUpgradeWarning=on
  Unit Delay1 : UnitDelay  Commented=through  SampleTime=-1  HasFrameUpgradeWarning=on
  Unit Delay2 : UnitDelay  Commented=through  SampleTime=-1  HasFrameUpgradeWarning=on
  x./D2 : Product
  xS2 : Product
  R2 : Outport
  x2 : Outport  Port=2
  wires:
  F2/1 -> Unit Delay1/1, Add1/1
  Divide1/1 -> x./D2/1
  Integrator1/1 -> x2/1, xS2/1
  x./D2/1 -> Integrator1/1
  Add1/1 -> Unit Delay/1, x./D2/2
  Constant3/1 -> Divide1/1
  R1/1 -> Add1/2
  S2/1 -> xS2/2
  Add/1 -> R2/1
  Unit Delay/1 -> Add/3
  xS2/1 -> Unit Delay2/1, Add1/3
  Unit Delay1/1 -> Add/1
  Unit Delay2/1 -> Add/2
  D2/1 -> Divide1/2

== system walkingRobotRL3D/Walking Robot/DYNAMIC MODEL OF PAM FOR LEFT LEG/Dynamic Model Antagonisitic PAM3/Spring and damping model/Dynamics muscle 1 ==
  F1 : Inport
  S1 : Inport  Port=2
  R2 : Inport  Port=3
  D1 : Inport  Port=4
  Add : Sum  Inputs=+--
  Add1 : Sum  Inputs=+--
  Constant1 : Constant
  Divide : Product  Inputs=*/
  Integrator : Integrator  InitialCondition=x10_ankleI_roll
  Unit Delay : UnitDelay  Commented=through  SampleTime=-1  HasFrameUpgradeWarning=on
  Unit Delay1 : UnitDelay  Commented=through  SampleTime=-1  HasFrameUpgradeWarning=on
  Unit Delay2 : UnitDelay  Commented=through  SampleTime=-1  HasFrameUpgradeWarning=on
  x./D1 : Product
  xS1 : Product
  R1 : Outport
  x1 : Outport  Port=2
  wires:
  Integrator/1 -> xS1/1, x1/1
  Divide/1 -> x./D1/1
  F1/1 -> Unit Delay1/1, Add/1
  x./D1/1 -> Integrator/1
  Add/1 -> Unit Delay/1, x./D1/2
  S1/1 -> xS1/2
  Constant1/1 -> Divide/1
  R2/1 -> Add/2
  Unit Delay/1 -> Add1/3
  Add1/1 -> R1/1
  xS1/1 -> Unit Delay2/1, Add/3
  D1/1 -> Divide/2
  Unit Delay1/1 -> Add1/1
  Unit Delay2/1 -> Add1/2

== system walkingRobotRL3D/Walking Robot/DYNAMIC MODEL OF PAM FOR LEFT LEG/Dynamic Model Antagonisitic PAM4/Spring and damping model/Dynamic muscle 2 ==
  S2 : Inport
  R1 : Inport  Port=2
  F2 : Inport  Port=3
  D2 : Inport  Port=4
  Add : Sum  Inputs=+--
  Add1 : Sum  Inputs=+--
  Constant3 : Constant
  Divide1 : Product  Inputs=*/
  Integrator1 : Integrator  InitialCondition=x20_hipI_roll
  Unit Delay : UnitDelay  Commented=through  SampleTime=-1  HasFrameUpgradeWarning=on
  Unit Delay1 : UnitDelay  Commented=through  SampleTime=-1  HasFrameUpgradeWarning=on
  Unit Delay2 : UnitDelay  Commented=through  SampleTime=-1  HasFrameUpgradeWarning=on
  x./D2 : Product
  xS2 : Product
  R2 : Outport
  x2 : Outport  Port=2
  wires:
  F2/1 -> Unit Delay1/1, Add1/1
  Divide1/1 -> x./D2/1
  Integrator1/1 -> x2/1, xS2/1
  x./D2/1 -> Integrator1/1
  Add1/1 -> Unit Delay/1, x./D2/2
  Constant3/1 -> Divide1/1
  R1/1 -> Add1/2
  S2/1 -> xS2/2
  Add/1 -> R2/1
  Unit Delay/1 -> Add/3
  xS2/1 -> Unit Delay2/1, Add1/3
  Unit Delay1/1 -> Add/1
  Unit Delay2/1 -> Add/2
  D2/1 -> Divide1/2

== system walkingRobotRL3D/Walking Robot/DYNAMIC MODEL OF PAM FOR LEFT LEG/Dynamic Model Antagonisitic PAM4/Spring and damping model/Dynamics muscle 1 ==
  F1 : Inport
  S1 : Inport  Port=2
  R2 : Inport  Port=3
  D1 : Inport  Port=4
  Add : Sum  Inputs=+--
  Add1 : Sum  Inputs=+--
  Constant1 : Constant
  Divide : Product  Inputs=*/
  Integrator : Integrator  InitialCondition=x10_hipI_roll
  Unit Delay : UnitDelay  Commented=through  SampleTime=-1  HasFrameUpgradeWarning=on
  Unit Delay1 : UnitDelay  Commented=through  SampleTime=-1  HasFrameUpgradeWarning=on
  Unit Delay2 : UnitDelay  Commented=through  SampleTime=-1  HasFrameUpgradeWarning=on
  x./D1 : Product
  xS1 : Product
  R1 : Outport
  x1 : Outport  Port=2
  wires:
  Integrator/1 -> xS1/1, x1/1
  Divide/1 -> x./D1/1
  F1/1 -> Unit Delay1/1, Add/1
  x./D1/1 -> Integrator/1
  Add/1 -> Unit Delay/1, x./D1/2
  S1/1 -> xS1/2
  Constant1/1 -> Divide/1
  R2/1 -> Add/2
  Unit Delay/1 -> Add1/3
  Add1/1 -> R1/1
  xS1/1 -> Unit Delay2/1, Add/3
  D1/1 -> Divide/2
  Unit Delay1/1 -> Add1/1
  Unit Delay2/1 -> Add1/2

== system walkingRobotRL3D/Walking Robot/DYNAMIC MODEL OF PAM FOR LEFT LEG/Dynamic Model Antagonisitic PAM5/Spring and damping model/Dynamic muscle 2 ==
  S2 : Inport
  R1 : Inport  Port=2
  F2 : Inport  Port=3
  D2 : Inport  Port=4
  Add : Sum  Inputs=+--
  Add1 : Sum  Inputs=+--
  Constant3 : Constant
  Divide1 : Product  Inputs=*/
  Integrator1 : Integrator  InitialCondition=x20_hipI_pitch
  Unit Delay : UnitDelay  Commented=through  SampleTime=-1  HasFrameUpgradeWarning=on
  Unit Delay1 : UnitDelay  Commented=through  SampleTime=-1  HasFrameUpgradeWarning=on
  Unit Delay2 : UnitDelay  Commented=through  SampleTime=-1  HasFrameUpgradeWarning=on
  x./D2 : Product
  xS2 : Product
  R2 : Outport
  x2 : Outport  Port=2
  wires:
  F2/1 -> Unit Delay1/1, Add1/1
  Divide1/1 -> x./D2/1
  Integrator1/1 -> x2/1, xS2/1
  x./D2/1 -> Integrator1/1
  Add1/1 -> Unit Delay/1, x./D2/2
  Constant3/1 -> Divide1/1
  R1/1 -> Add1/2
  S2/1 -> xS2/2
  Add/1 -> R2/1
  Unit Delay/1 -> Add/3
  xS2/1 -> Unit Delay2/1, Add1/3
  Unit Delay1/1 -> Add/1
  Unit Delay2/1 -> Add/2
  D2/1 -> Divide1/2

== system walkingRobotRL3D/Walking Robot/DYNAMIC MODEL OF PAM FOR LEFT LEG/Dynamic Model Antagonisitic PAM5/Spring and damping model/Dynamics muscle 1 ==
  F1 : Inport
  S1 : Inport  Port=2
  R2 : Inport  Port=3
  D1 : Inport  Port=4
  Add : Sum  Inputs=+--
  Add1 : Sum  Inputs=+--
  Constant1 : Constant
  Divide : Product  Inputs=*/
  Integrator : Integrator  InitialCondition=x10_hipI_pitch
  Unit Delay : UnitDelay  Commented=through  SampleTime=-1  HasFrameUpgradeWarning=on
  Unit Delay1 : UnitDelay  Commented=through  SampleTime=-1  HasFrameUpgradeWarning=on
  Unit Delay2 : UnitDelay  Commented=through  SampleTime=-1  HasFrameUpgradeWarning=on
  x./D1 : Product
  xS1 : Product
  R1 : Outport
  x1 : Outport  Port=2
  wires:
  Integrator/1 -> xS1/1, x1/1
  Divide/1 -> x./D1/1
  F1/1 -> Unit Delay1/1, Add/1
  x./D1/1 -> Integrator/1
  Add/1 -> Unit Delay/1, x./D1/2
  S1/1 -> xS1/2
  Constant1/1 -> Divide/1
  R2/1 -> Add/2
  Unit Delay/1 -> Add1/3
  Add1/1 -> R1/1
  xS1/1 -> Unit Delay2/1, Add/3
  D1/1 -> Divide/2
  Unit Delay1/1 -> Add1/1
  Unit Delay2/1 -> Add1/2

== system walkingRobotRL3D/Walking Robot/DYNAMIC MODEL OF PAM FOR RIGHT LEG/Dynamic Model Antagonisitic PAM1/Spring and damping model/Dynamic muscle 2 ==
  S2 : Inport
  R1 : Inport  Port=2
  F2 : Inport  Port=3
  D2 : Inport  Port=4
  Add : Sum  Inputs=+--
  Add1 : Sum  Inputs=+--
  Constant3 : Constant
  Divide1 : Product  Inputs=*/
  Integrator1 : Integrator  InitialCondition=x20_ankleD_pitch
  Unit Delay : UnitDelay  Commented=through  SampleTime=-1  HasFrameUpgradeWarning=on
  Unit Delay1 : UnitDelay  Commented=through  SampleTime=-1  HasFrameUpgradeWarning=on
  Unit Delay2 : UnitDelay  Commented=through  SampleTime=-1  HasFrameUpgradeWarning=on
  x./D2 : Product
  xS2 : Product
  R2 : Outport
  x2 : Outport  Port=2
  wires:
  F2/1 -> Unit Delay1/1, Add1/1
  Divide1/1 -> x./D2/1
  Integrator1/1 -> x2/1, xS2/1
  x./D2/1 -> Integrator1/1
  Add1/1 -> Unit Delay/1, x./D2/2
  Constant3/1 -> Divide1/1
  R1/1 -> Add1/2
  S2/1 -> xS2/2
  Add/1 -> R2/1
  Unit Delay/1 -> Add/3
  xS2/1 -> Unit Delay2/1, Add1/3
  Unit Delay1/1 -> Add/1
  Unit Delay2/1 -> Add/2
  D2/1 -> Divide1/2
